simulink model "Manchester"  (R2014a)
settings: Solver=ode45  StartTime=0.0  StopTime=10.0  RelTol=1e-3
settings Model: Creator=qiji  LastModifiedBy=qiji
settings DebuggingCC: UnderspecifiedInitializationDetection=Classic

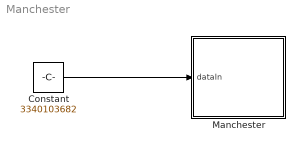
== system Manchester ==
  Constant : Constant  Value=3340103682  OutDataTypeStr=uint32
  Manchester : Stateflow chart  TreatAsAtomicUnit=on
  wires:
  Constant/1 -> Manchester/1(dataIn)

== stateflow chart Manchester/Manchester ==
  state start
  state end
  (default) -> start
  start -> end : {
      | dataOutEncoding = ManchesterEncoding(dataIn);
      | dataOutDecoding = ManchesterDecoding(dataOutEncoding);
      | }
  data: data function_input uint32; r function_output uint32; r function_output uint32; data function_input uint32; dataIn input uint32; dataOutEncoding local uint32; dataOutDecoding local double
  function r = ManchesterEncoding(data):
    | function r = ManchesterEncoding(data)
    | r = data;
    | for i = 1:16
    |     x = bitget(data, i);
    |     if x == 0
    |         r = bitset(r, i*2-1, 1);
    |         r = bitset(r, i*2, 0);
    |     else
    |         r = bitset(r, i*2-1, 0);
    |         r = bitset(r, i*2, 1);
    |     end
    | end
  function r = ManchesterDecoding(data):
    | function r = ManchesterDecoding(data)
    | r = data;
    | for i = (1:2:32)
    |     x0 = bitget(data, i);
    |     x1 = bitget(data, i+1);
    |     if x0==0 && x1==1
    |         r = bitset(r, (i+1)/2, 1);
    |     else
    |         r = bitset(r, (i+1)/2, 0);
    |     end
    | end
    | for i = (16:32)
    |     r = bitset(r, i, 0);
    | end
